simulink model "TST_DrvDem_SelectParameter"  (R2016b)
settings: Solver=FixedStepDiscrete  StartTime=0.0  StopTime=simTime  FixedStep=sampleTime  RelTol=1e-3
values from neighbouring files (symbols this model uses):
  testCase = 1    [initTST_DrvDem_SelectParameter_001.m]    (also in initTST_DrvDem_SelectParameter_002.m = 2; initTST_DrvDem_SelectParameter_003.m = 3)
libraries: simulink x82, UnitTest_Lib x78
(part 3 of 3)

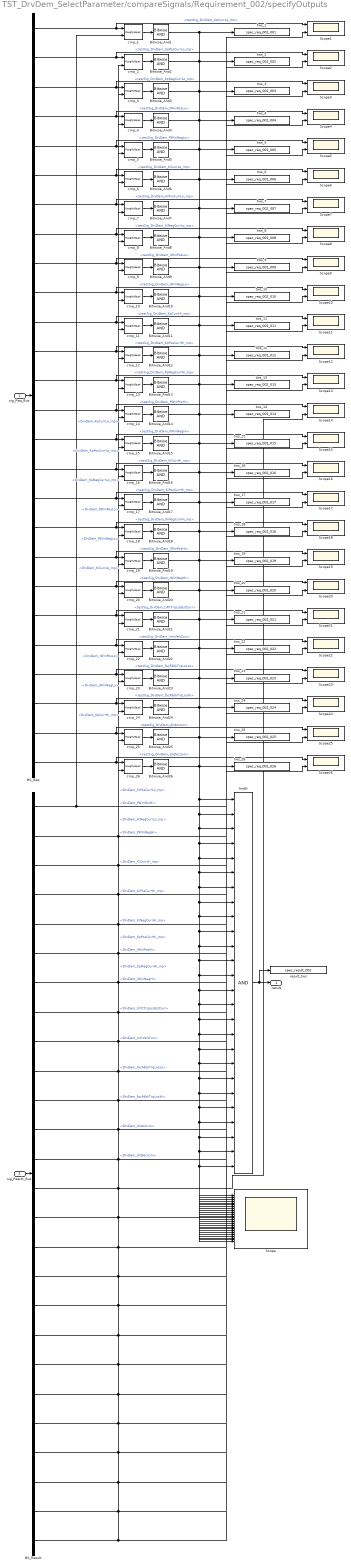
== system TST_DrvDem_SelectParameter/compareSignals/Requirement_002/specifyOutputs ==
  sig_Req_Bus : Inport
  sig_Result_Bus : Inport  Port=2
  AndN : Logic  Inputs=26
  BS_Req : BusSelector  OutputSignals=testSig_DrvDem_KpCurrLo_mp,testSig_DrvDem_KpPosCurrLo_mp,testSig_DrvDem_KpNegCurrLo_mp,testSig_DrvDem_PWinPosLo,testSig_DrvDem_PWinNegLo,testSig_DrvDem_KiCurrLo_mp,testSig_DrvDem_KiPosCurrLo_mp,testSig_DrvDem_KiNegCurrLo_mp,testSig_DrvDem_IWinPosLo,testSig_DrvDem_IWinNegLo,testSig_DrvDem_KpCurrHi_mp,testSig_DrvDem_KpPosCurrHi_mp,testSig_DrvDem_KpNegCurrHi_mp,testSig_DrvDem_PWinPosHi,testSig_DrvDem_PWinNegHi,testSig_DrvDem_KiCurrHi_mp,testSig_DrvDem_KiPosCurrHi_mp,testSig_DrvDem_KiNegCurrHi_mp,testSig_DrvDem_IWinPosHi,testSig_DrvDem_IWinNegHi,testSig_DrvDem_tiFltTrqLosEstCurr,testSig_DrvDem_InrtVehCurr,testSig_DrvDem_facFdbkTrqLosLo,testSig_DrvDem_facFdbkTrqLosHi,testSig_DrvDem_dnAccLim,testSig_DrvDem_dnDeclLim
  BS_Result : BusSelector  OutputSignals=DrvDem_KpCurrLo_mp,DrvDem_KpPosCurrLo_mp,DrvDem_KpNegCurrLo_mp,DrvDem_PWinPosLo,DrvDem_PWinNegLo,DrvDem_KiCurrLo_mp,DrvDem_KiPosCurrLo_mp,DrvDem_KiNegCurrLo_mp,DrvDem_IWinPosLo,DrvDem_IWinNegLo,DrvDem_KpCurrHi_mp,DrvDem_KpPosCurrHi_mp,DrvDem_KpNegCurrHi_mp,DrvDem_PWinPosHi,DrvDem_PWinNegHi,DrvDem_KiCurrHi_mp,DrvDem_KiPosCurrHi_mp,DrvDem_KiNegCurrHi_mp,DrvDem_IWinPosHi,DrvDem_IWinNegHi,DrvDem_tiFltTrqLosEstCurr,DrvDem_InrtVehCurr,DrvDem_facFdbkTrqLosLo,DrvDem_facFdbkTrqLosHi,DrvDem_dnAccLim,DrvDem_dnDeclLim
  Bitwise_And{1..26} (26 alike) : simulink/Logic and Bit Operations/Bitwise Operator  logicop=AND  UseBitMask=off  BitMask=bin2dec('11011001')  BitMaskRealWorld=Stored Integer
  Scope : Scope  NumInputPorts=26
  Scope{1..26} (26 alike) : Scope  NumInputPorts=2
  cmp_{1..24} (24 alike) : UnitTest_Lib/RoughlyEqual  slope=0.1
  cmp_25 : UnitTest_Lib/RoughlyEqual  slope=1
  cmp_26 : UnitTest_Lib/RoughlyEqual  slope=1
  result_tws : ToWorkspace  VariableName=spec_result_002
  tws_1 : ToWorkspace  VariableName=spec_req_002_001
  tws_10 : ToWorkspace  VariableName=spec_req_002_010
  tws_11 : ToWorkspace  VariableName=spec_req_002_011
  tws_12 : ToWorkspace  VariableName=spec_req_002_012
  tws_13 : ToWorkspace  VariableName=spec_req_002_013
  tws_14 : ToWorkspace  VariableName=spec_req_002_014
  tws_15 : ToWorkspace  VariableName=spec_req_002_015
  tws_16 : ToWorkspace  VariableName=spec_req_002_016
  tws_17 : ToWorkspace  VariableName=spec_req_002_017
  tws_18 : ToWorkspace  VariableName=spec_req_002_018
  tws_19 : ToWorkspace  VariableName=spec_req_002_019
  tws_2 : ToWorkspace  VariableName=spec_req_002_002
  tws_20 : ToWorkspace  VariableName=spec_req_002_020
  tws_21 : ToWorkspace  VariableName=spec_req_002_021
  tws_22 : ToWorkspace  VariableName=spec_req_002_022
  tws_23 : ToWorkspace  VariableName=spec_req_002_023
  tws_24 : ToWorkspace  VariableName=spec_req_002_024
  tws_25 : ToWorkspace  VariableName=spec_req_002_025
  tws_26 : ToWorkspace  VariableName=spec_req_002_026
  tws_3 : ToWorkspace  VariableName=spec_req_002_003
  tws_4 : ToWorkspace  VariableName=spec_req_002_004
  tws_5 : ToWorkspace  VariableName=spec_req_002_005
  tws_6 : ToWorkspace  VariableName=spec_req_002_006
  tws_7 : ToWorkspace  VariableName=spec_req_002_007
  tws_8 : ToWorkspace  VariableName=spec_req_002_008
  tws_9 : ToWorkspace  VariableName=spec_req_002_009
  result : Outport
  wires:
  sig_Req_Bus/1 -> BS_Req/1
  sig_Result_Bus/1 -> BS_Result/1
  AndN/1 -> result/1, result_tws/1
  BS_Req/1 -> cmp_1/1, Scope1/1  "<testSig_DrvDem_KpCurrLo_mp>"
  BS_Result/1 -> cmp_1/2, Scope1/2  "<DrvDem_KpCurrLo_mp>"
  cmp_1/1 -> Bitwise_And1/1
  Bitwise_And1/1 -> AndN/1, Scope/1, tws_1/1
  BS_Req/2 -> cmp_2/1, Scope2/1  "<testSig_DrvDem_KpPosCurrLo_mp>"
  BS_Result/2 -> cmp_2/2, Scope2/2  "<DrvDem_KpPosCurrLo_mp>"
  cmp_2/1 -> Bitwise_And2/1
  Bitwise_And2/1 -> AndN/2, Scope/2, tws_2/1
  BS_Req/3 -> cmp_3/1, Scope3/1  "<testSig_DrvDem_KpNegCurrLo_mp>"
  BS_Result/3 -> cmp_3/2, Scope3/2  "<DrvDem_KpNegCurrLo_mp>"
  cmp_3/1 -> Bitwise_And3/1
  Bitwise_And3/1 -> AndN/3, Scope/3, tws_3/1
  BS_Req/4 -> cmp_4/1, Scope4/1  "<testSig_DrvDem_PWinPosLo>"
  BS_Result/4 -> cmp_4/2, Scope4/2  "<DrvDem_PWinPosLo>"
  cmp_4/1 -> Bitwise_And4/1
  Bitwise_And4/1 -> AndN/4, Scope/4, tws_4/1
  BS_Req/5 -> cmp_5/1, Scope5/1  "<testSig_DrvDem_PWinNegLo>"
  BS_Result/5 -> cmp_5/2, Scope5/2  "<DrvDem_PWinNegLo>"
  cmp_5/1 -> Bitwise_And5/1
  Bitwise_And5/1 -> AndN/5, Scope/5, tws_5/1
  BS_Req/6 -> cmp_6/1, Scope6/1  "<testSig_DrvDem_KiCurrLo_mp>"
  BS_Result/6 -> cmp_6/2, Scope6/2  "<DrvDem_KiCurrLo_mp>"
  cmp_6/1 -> Bitwise_And6/1
  Bitwise_And6/1 -> AndN/6, Scope/6, tws_6/1
  BS_Req/7 -> cmp_7/1, Scope7/1  "<testSig_DrvDem_KiPosCurrLo_mp>"
  BS_Result/7 -> cmp_7/2, Scope7/2  "<DrvDem_KiPosCurrLo_mp>"
  cmp_7/1 -> Bitwise_And7/1
  Bitwise_And7/1 -> AndN/7, Scope/7, tws_7/1
  BS_Req/8 -> cmp_8/1, Scope8/1  "<testSig_DrvDem_KiNegCurrLo_mp>"
  BS_Result/8 -> cmp_8/2, Scope8/2  "<DrvDem_KiNegCurrLo_mp>"
  cmp_8/1 -> Bitwise_And8/1
  Bitwise_And8/1 -> AndN/8, Scope/8, tws_8/1
  BS_Req/9 -> cmp_9/1, Scope9/1  "<testSig_DrvDem_IWinPosLo>"
  BS_Result/9 -> cmp_9/2, Scope9/2  "<DrvDem_IWinPosLo>"
  cmp_9/1 -> Bitwise_And9/1
  Bitwise_And9/1 -> AndN/9, Scope/9, tws_9/1
  BS_Req/10 -> cmp_10/1, Scope10/1  "<testSig_DrvDem_IWinNegLo>"
  BS_Result/10 -> cmp_10/2, Scope10/2  "<DrvDem_IWinNegLo>"
  cmp_10/1 -> Bitwise_And10/1
  Bitwise_And10/1 -> AndN/10, Scope/10, tws_10/1
  BS_Req/11 -> cmp_11/1, Scope11/1  "<testSig_DrvDem_KpCurrHi_mp>"
  BS_Result/11 -> cmp_11/2, Scope11/2  "<DrvDem_KpCurrHi_mp>"
  cmp_11/1 -> Bitwise_And11/1
  Bitwise_And11/1 -> AndN/11, Scope/11, tws_11/1
  BS_Req/12 -> cmp_12/1, Scope12/1  "<testSig_DrvDem_KpPosCurrHi_mp>"
  BS_Result/12 -> cmp_12/2, Scope12/2  "<DrvDem_KpPosCurrHi_mp>"
  cmp_12/1 -> Bitwise_And12/1
  Bitwise_And12/1 -> AndN/12, Scope/12, tws_12/1
  BS_Req/13 -> cmp_13/1, Scope13/1  "<testSig_DrvDem_KpNegCurrHi_mp>"
  BS_Result/13 -> cmp_13/2, Scope13/2  "<DrvDem_KpNegCurrHi_mp>"
  cmp_13/1 -> Bitwise_And13/1
  Bitwise_And13/1 -> AndN/13, Scope/13, tws_13/1
  BS_Req/14 -> cmp_14/1, Scope14/1  "<testSig_DrvDem_PWinPosHi>"
  BS_Result/14 -> cmp_14/2, Scope14/2  "<DrvDem_PWinPosHi>"
  cmp_14/1 -> Bitwise_And14/1
  Bitwise_And14/1 -> AndN/14, Scope/14, tws_14/1
  BS_Req/15 -> cmp_15/1, Scope15/1  "<testSig_DrvDem_PWinNegHi>"
  BS_Result/15 -> cmp_15/2, Scope15/2  "<DrvDem_PWinNegHi>"
  cmp_15/1 -> Bitwise_And15/1
  Bitwise_And15/1 -> AndN/15, Scope/15, tws_15/1
  BS_Req/16 -> cmp_16/1, Scope16/1  "<testSig_DrvDem_KiCurrHi_mp>"
  BS_Result/16 -> cmp_16/2, Scope16/2  "<DrvDem_KiCurrHi_mp>"
  cmp_16/1 -> Bitwise_And16/1
  Bitwise_And16/1 -> AndN/16, Scope/16, tws_16/1
  BS_Req/17 -> cmp_17/1, Scope17/1  "<testSig_DrvDem_KiPosCurrHi_mp>"
  BS_Result/17 -> cmp_17/2, Scope17/2  "<DrvDem_KiPosCurrHi_mp>"
  cmp_17/1 -> Bitwise_And17/1
  Bitwise_And17/1 -> AndN/17, Scope/17, tws_17/1
  BS_Req/18 -> cmp_18/1, Scope18/1  "<testSig_DrvDem_KiNegCurrHi_mp>"
  BS_Result/18 -> cmp_18/2, Scope18/2  "<DrvDem_KiNegCurrHi_mp>"
  cmp_18/1 -> Bitwise_And18/1
  Bitwise_And18/1 -> AndN/18, Scope/18, tws_18/1
  BS_Req/19 -> cmp_19/1, Scope19/1  "<testSig_DrvDem_IWinPosHi>"
  BS_Result/19 -> cmp_19/2, Scope19/2  "<DrvDem_IWinPosHi>"
  cmp_19/1 -> Bitwise_And19/1
  Bitwise_And19/1 -> AndN/19, Scope/19, tws_19/1
  BS_Req/20 -> cmp_20/1, Scope20/1  "<testSig_DrvDem_IWinNegHi>"
  BS_Result/20 -> cmp_20/2, Scope20/2  "<DrvDem_IWinNegHi>"
  cmp_20/1 -> Bitwise_And20/1
  Bitwise_And20/1 -> AndN/20, Scope/20, tws_20/1
  BS_Req/21 -> cmp_21/1, Scope21/1  "<testSig_DrvDem_tiFltTrqLosEstCurr>"
  BS_Result/21 -> cmp_21/2, Scope21/2  "<DrvDem_tiFltTrqLosEstCurr>"
  cmp_21/1 -> Bitwise_And21/1
  Bitwise_And21/1 -> AndN/21, Scope/21, tws_21/1
  BS_Req/22 -> cmp_22/1, Scope22/1  "<testSig_DrvDem_InrtVehCurr>"
  BS_Result/22 -> cmp_22/2, Scope22/2  "<DrvDem_InrtVehCurr>"
  cmp_22/1 -> Bitwise_And22/1
  Bitwise_And22/1 -> AndN/22, Scope/22, tws_22/1
  BS_Req/23 -> cmp_23/1, Scope23/1  "<testSig_DrvDem_facFdbkTrqLosLo>"
  BS_Result/23 -> cmp_23/2, Scope23/2  "<DrvDem_facFdbkTrqLosLo>"
  cmp_23/1 -> Bitwise_And23/1
  Bitwise_And23/1 -> AndN/23, Scope/23, tws_23/1
  BS_Req/24 -> cmp_24/1, Scope24/1  "<testSig_DrvDem_facFdbkTrqLosHi>"
  BS_Result/24 -> cmp_24/2, Scope24/2  "<DrvDem_facFdbkTrqLosHi>"
  cmp_24/1 -> Bitwise_And24/1
  Bitwise_And24/1 -> AndN/24, Scope/24, tws_24/1
  BS_Req/25 -> cmp_25/1, Scope25/1  "<testSig_DrvDem_dnAccLim>"
  BS_Result/25 -> cmp_25/2, Scope25/2  "<DrvDem_dnAccLim>"
  cmp_25/1 -> Bitwise_And25/1
  Bitwise_And25/1 -> AndN/25, Scope/25, tws_25/1
  BS_Req/26 -> cmp_26/1, Scope26/1  "<testSig_DrvDem_dnDeclLim>"
  BS_Result/26 -> cmp_26/2, Scope26/2  "<DrvDem_dnDeclLim>"
  cmp_26/1 -> Bitwise_And26/1
  Bitwise_And26/1 -> AndN/26, Scope/26, tws_26/1

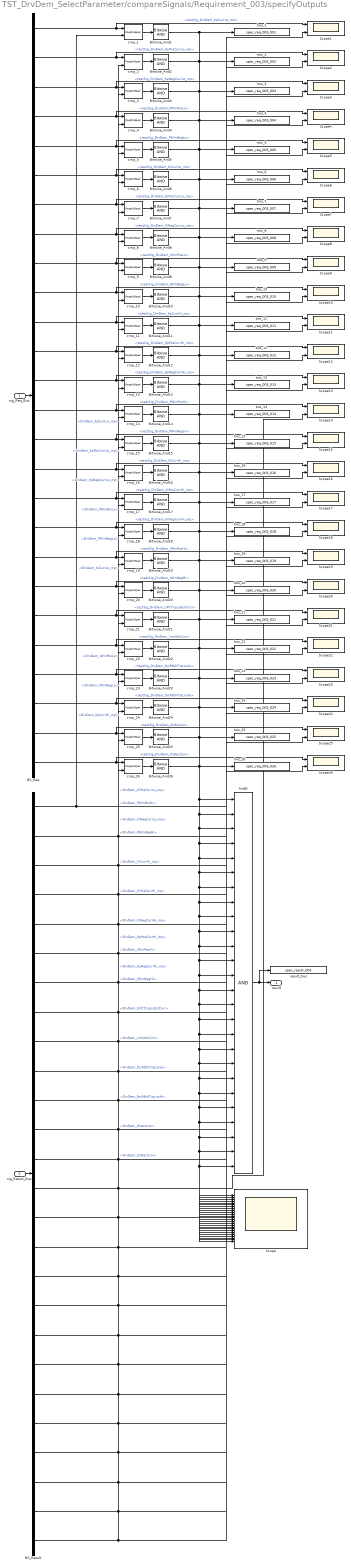
== system TST_DrvDem_SelectParameter/compareSignals/Requirement_003/specifyOutputs ==
  sig_Req_Bus : Inport
  sig_Result_Bus : Inport  Port=2
  AndN : Logic  Inputs=26
  BS_Req : BusSelector  OutputSignals=testSig_DrvDem_KpCurrLo_mp,testSig_DrvDem_KpPosCurrLo_mp,testSig_DrvDem_KpNegCurrLo_mp,testSig_DrvDem_PWinPosLo,testSig_DrvDem_PWinNegLo,testSig_DrvDem_KiCurrLo_mp,testSig_DrvDem_KiPosCurrLo_mp,testSig_DrvDem_KiNegCurrLo_mp,testSig_DrvDem_IWinPosLo,testSig_DrvDem_IWinNegLo,testSig_DrvDem_KpCurrHi_mp,testSig_DrvDem_KpPosCurrHi_mp,testSig_DrvDem_KpNegCurrHi_mp,testSig_DrvDem_PWinPosHi,testSig_DrvDem_PWinNegHi,testSig_DrvDem_KiCurrHi_mp,testSig_DrvDem_KiPosCurrHi_mp,testSig_DrvDem_KiNegCurrHi_mp,testSig_DrvDem_IWinPosHi,testSig_DrvDem_IWinNegHi,testSig_DrvDem_tiFltTrqLosEstCurr,testSig_DrvDem_InrtVehCurr,testSig_DrvDem_facFdbkTrqLosLo,testSig_DrvDem_facFdbkTrqLosHi,testSig_DrvDem_dnAccLim,testSig_DrvDem_dnDeclLim
  BS_Result : BusSelector  OutputSignals=DrvDem_KpCurrLo_mp,DrvDem_KpPosCurrLo_mp,DrvDem_KpNegCurrLo_mp,DrvDem_PWinPosLo,DrvDem_PWinNegLo,DrvDem_KiCurrLo_mp,DrvDem_KiPosCurrLo_mp,DrvDem_KiNegCurrLo_mp,DrvDem_IWinPosLo,DrvDem_IWinNegLo,DrvDem_KpCurrHi_mp,DrvDem_KpPosCurrHi_mp,DrvDem_KpNegCurrHi_mp,DrvDem_PWinPosHi,DrvDem_PWinNegHi,DrvDem_KiCurrHi_mp,DrvDem_KiPosCurrHi_mp,DrvDem_KiNegCurrHi_mp,DrvDem_IWinPosHi,DrvDem_IWinNegHi,DrvDem_tiFltTrqLosEstCurr,DrvDem_InrtVehCurr,DrvDem_facFdbkTrqLosLo,DrvDem_facFdbkTrqLosHi,DrvDem_dnAccLim,DrvDem_dnDeclLim
  Bitwise_And{1..26} (26 alike) : simulink/Logic and Bit Operations/Bitwise Operator  logicop=AND  UseBitMask=off  BitMask=bin2dec('11011001')  BitMaskRealWorld=Stored Integer
  Scope : Scope  NumInputPorts=26
  Scope{1..26} (26 alike) : Scope  NumInputPorts=2
  cmp_{1..24} (24 alike) : UnitTest_Lib/RoughlyEqual  slope=0.1
  cmp_25 : UnitTest_Lib/RoughlyEqual  slope=1
  cmp_26 : UnitTest_Lib/RoughlyEqual  slope=1
  result_tws : ToWorkspace  VariableName=spec_result_003
  tws_1 : ToWorkspace  VariableName=spec_req_003_001
  tws_10 : ToWorkspace  VariableName=spec_req_003_010
  tws_11 : ToWorkspace  VariableName=spec_req_003_011
  tws_12 : ToWorkspace  VariableName=spec_req_003_012
  tws_13 : ToWorkspace  VariableName=spec_req_003_013
  tws_14 : ToWorkspace  VariableName=spec_req_003_014
  tws_15 : ToWorkspace  VariableName=spec_req_003_015
  tws_16 : ToWorkspace  VariableName=spec_req_003_016
  tws_17 : ToWorkspace  VariableName=spec_req_003_017
  tws_18 : ToWorkspace  VariableName=spec_req_003_018
  tws_19 : ToWorkspace  VariableName=spec_req_003_019
  tws_2 : ToWorkspace  VariableName=spec_req_003_002
  tws_20 : ToWorkspace  VariableName=spec_req_003_020
  tws_21 : ToWorkspace  VariableName=spec_req_003_021
  tws_22 : ToWorkspace  VariableName=spec_req_003_022
  tws_23 : ToWorkspace  VariableName=spec_req_003_023
  tws_24 : ToWorkspace  VariableName=spec_req_003_024
  tws_25 : ToWorkspace  VariableName=spec_req_003_025
  tws_26 : ToWorkspace  VariableName=spec_req_003_026
  tws_3 : ToWorkspace  VariableName=spec_req_003_003
  tws_4 : ToWorkspace  VariableName=spec_req_003_004
  tws_5 : ToWorkspace  VariableName=spec_req_003_005
  tws_6 : ToWorkspace  VariableName=spec_req_003_006
  tws_7 : ToWorkspace  VariableName=spec_req_003_007
  tws_8 : ToWorkspace  VariableName=spec_req_003_008
  tws_9 : ToWorkspace  VariableName=spec_req_003_009
  result : Outport
  wires:
  sig_Req_Bus/1 -> BS_Req/1
  sig_Result_Bus/1 -> BS_Result/1
  AndN/1 -> result/1, result_tws/1
  BS_Req/1 -> cmp_1/1, Scope1/1  "<testSig_DrvDem_KpCurrLo_mp>"
  BS_Result/1 -> cmp_1/2, Scope1/2  "<DrvDem_KpCurrLo_mp>"
  cmp_1/1 -> Bitwise_And1/1
  Bitwise_And1/1 -> AndN/1, Scope/1, tws_1/1
  BS_Req/2 -> cmp_2/1, Scope2/1  "<testSig_DrvDem_KpPosCurrLo_mp>"
  BS_Result/2 -> cmp_2/2, Scope2/2  "<DrvDem_KpPosCurrLo_mp>"
  cmp_2/1 -> Bitwise_And2/1
  Bitwise_And2/1 -> AndN/2, Scope/2, tws_2/1
  BS_Req/3 -> cmp_3/1, Scope3/1  "<testSig_DrvDem_KpNegCurrLo_mp>"
  BS_Result/3 -> cmp_3/2, Scope3/2  "<DrvDem_KpNegCurrLo_mp>"
  cmp_3/1 -> Bitwise_And3/1
  Bitwise_And3/1 -> AndN/3, Scope/3, tws_3/1
  BS_Req/4 -> cmp_4/1, Scope4/1  "<testSig_DrvDem_PWinPosLo>"
  BS_Result/4 -> cmp_4/2, Scope4/2  "<DrvDem_PWinPosLo>"
  cmp_4/1 -> Bitwise_And4/1
  Bitwise_And4/1 -> AndN/4, Scope/4, tws_4/1
  BS_Req/5 -> cmp_5/1, Scope5/1  "<testSig_DrvDem_PWinNegLo>"
  BS_Result/5 -> cmp_5/2, Scope5/2  "<DrvDem_PWinNegLo>"
  cmp_5/1 -> Bitwise_And5/1
  Bitwise_And5/1 -> AndN/5, Scope/5, tws_5/1
  BS_Req/6 -> cmp_6/1, Scope6/1  "<testSig_DrvDem_KiCurrLo_mp>"
  BS_Result/6 -> cmp_6/2, Scope6/2  "<DrvDem_KiCurrLo_mp>"
  cmp_6/1 -> Bitwise_And6/1
  Bitwise_And6/1 -> AndN/6, Scope/6, tws_6/1
  BS_Req/7 -> cmp_7/1, Scope7/1  "<testSig_DrvDem_KiPosCurrLo_mp>"
  BS_Result/7 -> cmp_7/2, Scope7/2  "<DrvDem_KiPosCurrLo_mp>"
  cmp_7/1 -> Bitwise_And7/1
  Bitwise_And7/1 -> AndN/7, Scope/7, tws_7/1
  BS_Req/8 -> cmp_8/1, Scope8/1  "<testSig_DrvDem_KiNegCurrLo_mp>"
  BS_Result/8 -> cmp_8/2, Scope8/2  "<DrvDem_KiNegCurrLo_mp>"
  cmp_8/1 -> Bitwise_And8/1
  Bitwise_And8/1 -> AndN/8, Scope/8, tws_8/1
  BS_Req/9 -> cmp_9/1, Scope9/1  "<testSig_DrvDem_IWinPosLo>"
  BS_Result/9 -> cmp_9/2, Scope9/2  "<DrvDem_IWinPosLo>"
  cmp_9/1 -> Bitwise_And9/1
  Bitwise_And9/1 -> AndN/9, Scope/9, tws_9/1
  BS_Req/10 -> cmp_10/1, Scope10/1  "<testSig_DrvDem_IWinNegLo>"
  BS_Result/10 -> cmp_10/2, Scope10/2  "<DrvDem_IWinNegLo>"
  cmp_10/1 -> Bitwise_And10/1
  Bitwise_And10/1 -> AndN/10, Scope/10, tws_10/1
  BS_Req/11 -> cmp_11/1, Scope11/1  "<testSig_DrvDem_KpCurrHi_mp>"
  BS_Result/11 -> cmp_11/2, Scope11/2  "<DrvDem_KpCurrHi_mp>"
  cmp_11/1 -> Bitwise_And11/1
  Bitwise_And11/1 -> AndN/11, Scope/11, tws_11/1
  BS_Req/12 -> cmp_12/1, Scope12/1  "<testSig_DrvDem_KpPosCurrHi_mp>"
  BS_Result/12 -> cmp_12/2, Scope12/2  "<DrvDem_KpPosCurrHi_mp>"
  cmp_12/1 -> Bitwise_And12/1
  Bitwise_And12/1 -> AndN/12, Scope/12, tws_12/1
  BS_Req/13 -> cmp_13/1, Scope13/1  "<testSig_DrvDem_KpNegCurrHi_mp>"
  BS_Result/13 -> cmp_13/2, Scope13/2  "<DrvDem_KpNegCurrHi_mp>"
  cmp_13/1 -> Bitwise_And13/1
  Bitwise_And13/1 -> AndN/13, Scope/13, tws_13/1
  BS_Req/14 -> cmp_14/1, Scope14/1  "<testSig_DrvDem_PWinPosHi>"
  BS_Result/14 -> cmp_14/2, Scope14/2  "<DrvDem_PWinPosHi>"
  cmp_14/1 -> Bitwise_And14/1
  Bitwise_And14/1 -> AndN/14, Scope/14, tws_14/1
  BS_Req/15 -> cmp_15/1, Scope15/1  "<testSig_DrvDem_PWinNegHi>"
  BS_Result/15 -> cmp_15/2, Scope15/2  "<DrvDem_PWinNegHi>"
  cmp_15/1 -> Bitwise_And15/1
  Bitwise_And15/1 -> AndN/15, Scope/15, tws_15/1
  BS_Req/16 -> cmp_16/1, Scope16/1  "<testSig_DrvDem_KiCurrHi_mp>"
  BS_Result/16 -> cmp_16/2, Scope16/2  "<DrvDem_KiCurrHi_mp>"
  cmp_16/1 -> Bitwise_And16/1
  Bitwise_And16/1 -> AndN/16, Scope/16, tws_16/1
  BS_Req/17 -> cmp_17/1, Scope17/1  "<testSig_DrvDem_KiPosCurrHi_mp>"
  BS_Result/17 -> cmp_17/2, Scope17/2  "<DrvDem_KiPosCurrHi_mp>"
  cmp_17/1 -> Bitwise_And17/1
  Bitwise_And17/1 -> AndN/17, Scope/17, tws_17/1
  BS_Req/18 -> cmp_18/1, Scope18/1  "<testSig_DrvDem_KiNegCurrHi_mp>"
  BS_Result/18 -> cmp_18/2, Scope18/2  "<DrvDem_KiNegCurrHi_mp>"
  cmp_18/1 -> Bitwise_And18/1
  Bitwise_And18/1 -> AndN/18, Scope/18, tws_18/1
  BS_Req/19 -> cmp_19/1, Scope19/1  "<testSig_DrvDem_IWinPosHi>"
  BS_Result/19 -> cmp_19/2, Scope19/2  "<DrvDem_IWinPosHi>"
  cmp_19/1 -> Bitwise_And19/1
  Bitwise_And19/1 -> AndN/19, Scope/19, tws_19/1
  BS_Req/20 -> cmp_20/1, Scope20/1  "<testSig_DrvDem_IWinNegHi>"
  BS_Result/20 -> cmp_20/2, Scope20/2  "<DrvDem_IWinNegHi>"
  cmp_20/1 -> Bitwise_And20/1
  Bitwise_And20/1 -> AndN/20, Scope/20, tws_20/1
  BS_Req/21 -> cmp_21/1, Scope21/1  "<testSig_DrvDem_tiFltTrqLosEstCurr>"
  BS_Result/21 -> cmp_21/2, Scope21/2  "<DrvDem_tiFltTrqLosEstCurr>"
  cmp_21/1 -> Bitwise_And21/1
  Bitwise_And21/1 -> AndN/21, Scope/21, tws_21/1
  BS_Req/22 -> cmp_22/1, Scope22/1  "<testSig_DrvDem_InrtVehCurr>"
  BS_Result/22 -> cmp_22/2, Scope22/2  "<DrvDem_InrtVehCurr>"
  cmp_22/1 -> Bitwise_And22/1
  Bitwise_And22/1 -> AndN/22, Scope/22, tws_22/1
  BS_Req/23 -> cmp_23/1, Scope23/1  "<testSig_DrvDem_facFdbkTrqLosLo>"
  BS_Result/23 -> cmp_23/2, Scope23/2  "<DrvDem_facFdbkTrqLosLo>"
  cmp_23/1 -> Bitwise_And23/1
  Bitwise_And23/1 -> AndN/23, Scope/23, tws_23/1
  BS_Req/24 -> cmp_24/1, Scope24/1  "<testSig_DrvDem_facFdbkTrqLosHi>"
  BS_Result/24 -> cmp_24/2, Scope24/2  "<DrvDem_facFdbkTrqLosHi>"
  cmp_24/1 -> Bitwise_And24/1
  Bitwise_And24/1 -> AndN/24, Scope/24, tws_24/1
  BS_Req/25 -> cmp_25/1, Scope25/1  "<testSig_DrvDem_dnAccLim>"
  BS_Result/25 -> cmp_25/2, Scope25/2  "<DrvDem_dnAccLim>"
  cmp_25/1 -> Bitwise_And25/1
  Bitwise_And25/1 -> AndN/25, Scope/25, tws_25/1
  BS_Req/26 -> cmp_26/1, Scope26/1  "<testSig_DrvDem_dnDeclLim>"
  BS_Result/26 -> cmp_26/2, Scope26/2  "<DrvDem_dnDeclLim>"
  cmp_26/1 -> Bitwise_And26/1
  Bitwise_And26/1 -> AndN/26, Scope/26, tws_26/1
